simulink subsystem "InjectorPablo"  (R2020b)
settings: Solver=VariableStepAuto  StartTime=0.0  StopTime=10.0  RelTol=1e-3
model mask{centerHolesDiam=0.89e-3, edgeHolesDiam=0.63e-3}
  mask prompts: centerHolesDiam "Center holes diameter (m)"; edgeHolesDiam "Edge holes diameter (m)"
libraries: fl_lib x8, nesl_utility x2
settings Model: Creator=Edward  LastModifiedBy=Edward

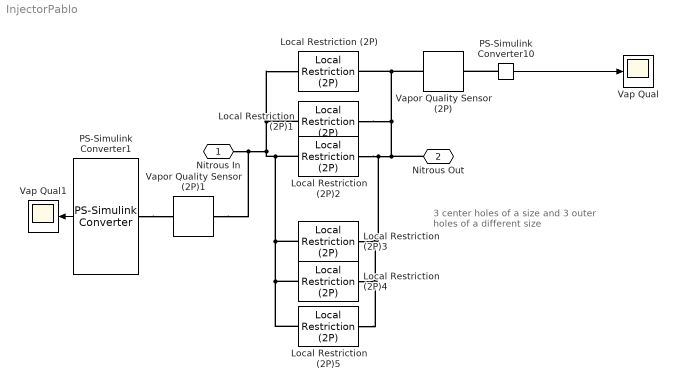
== system InjectorPablo ==
  note: 3 center holes of a size
      | and 3 outer holes of a different size
  Local Restriction (2P) : fl_lib/Two-Phase Fluid/Elements/Local Restriction (2P)  restriction_area=0.25.*pi.*centerHolesDiam.^2 m^2  area=Sim.preInjectorPipe.crossSection m^2  Cd=0.64  B_lam=0.999
      settings: SourceProductBaseCode=SS  InternalSimscapePortConfiguration="{\"Bottom\":[],\"Left\":[{\"id\":\"A\",\"label\":\"A\",\"type\":\"foundation.two_phase_fluid.two_phase_fluid\"}],\"Right\":[{\"id\":\"B\",\"label\":\"B\",\"type\":\"foundation.two_phase_fluid.two_phase_fluid\"}],\"Top\":[]}"
  Local Restriction (2P)1 : fl_lib/Two-Phase Fluid/Elements/Local Restriction (2P)  restriction_area=0.25.*pi.*centerHolesDiam.^2 m^2  area=Sim.preInjectorPipe.crossSection m^2  Cd=0.64  B_lam=0.999
      settings: SourceProductBaseCode=SS  InternalSimscapePortConfiguration="{\"Bottom\":[],\"Left\":[{\"id\":\"A\",\"label\":\"A\",\"type\":\"foundation.two_phase_fluid.two_phase_fluid\"}],\"Right\":[{\"id\":\"B\",\"label\":\"B\",\"type\":\"foundation.two_phase_fluid.two_phase_fluid\"}],\"Top\":[]}"
  Local Restriction (2P)2 : fl_lib/Two-Phase Fluid/Elements/Local Restriction (2P)  restriction_area=0.25.*pi.*centerHolesDiam.^2 m^2  area=Sim.preInjectorPipe.crossSection m^2  Cd=0.64  B_lam=0.999
      settings: SourceProductBaseCode=SS  InternalSimscapePortConfiguration="{\"Bottom\":[],\"Left\":[{\"id\":\"A\",\"label\":\"A\",\"type\":\"foundation.two_phase_fluid.two_phase_fluid\"}],\"Right\":[{\"id\":\"B\",\"label\":\"B\",\"type\":\"foundation.two_phase_fluid.two_phase_fluid\"}],\"Top\":[]}"
  Local Restriction (2P)3 : fl_lib/Two-Phase Fluid/Elements/Local Restriction (2P)  restriction_area=0.25.*pi.*edgeHolesDiam.^2 m^2  area=Sim.preInjectorPipe.crossSection m^2  Cd=0.64  B_lam=0.999
      settings: SourceProductBaseCode=SS  InternalSimscapePortConfiguration="{\"Bottom\":[],\"Left\":[{\"id\":\"A\",\"label\":\"A\",\"type\":\"foundation.two_phase_fluid.two_phase_fluid\"}],\"Right\":[{\"id\":\"B\",\"label\":\"B\",\"type\":\"foundation.two_phase_fluid.two_phase_fluid\"}],\"Top\":[]}"
  Local Restriction (2P)4 : fl_lib/Two-Phase Fluid/Elements/Local Restriction (2P)  restriction_area=0.25.*pi.*edgeHolesDiam.^2 m^2  area=Sim.preInjectorPipe.crossSection m^2  Cd=0.64  B_lam=0.999
      settings: SourceProductBaseCode=SS  InternalSimscapePortConfiguration="{\"Bottom\":[],\"Left\":[{\"id\":\"A\",\"label\":\"A\",\"type\":\"foundation.two_phase_fluid.two_phase_fluid\"}],\"Right\":[{\"id\":\"B\",\"label\":\"B\",\"type\":\"foundation.two_phase_fluid.two_phase_fluid\"}],\"Top\":[]}"
  Local Restriction (2P)5 : fl_lib/Two-Phase Fluid/Elements/Local Restriction (2P)  restriction_area=0.25.*pi.*edgeHolesDiam.^2 m^2  area=Sim.preInjectorPipe.crossSection m^2  Cd=0.64  B_lam=0.999
      settings: SourceProductBaseCode=SS  InternalSimscapePortConfiguration="{\"Bottom\":[],\"Left\":[{\"id\":\"A\",\"label\":\"A\",\"type\":\"foundation.two_phase_fluid.two_phase_fluid\"}],\"Right\":[{\"id\":\"B\",\"label\":\"B\",\"type\":\"foundation.two_phase_fluid.two_phase_fluid\"}],\"Top\":[]}"
  PS-Simulink Converter1 : nesl_utility/PS-Simulink Converter  PhysicalDomain=network_engine_domain  SubClassName=ps_output  LeftPortType=input  RightPortType=output  PseudoPeriodic=off  Frequencies=[]  Unit=inherit  AffineConversion=off
  PS-Simulink Converter10 : nesl_utility/PS-Simulink Converter  PhysicalDomain=network_engine_domain  SubClassName=ps_output  LeftPortType=input  RightPortType=output  PseudoPeriodic=off  Frequencies=[]  Unit=inherit  AffineConversion=off
  Vap Qual : Scope
  Vap Qual1 : Scope
  Vapor Quality Sensor (2P) : fl_lib/Two-Phase Fluid/Sensors/Vapor Quality Sensor (2P)  vapor_fraction_spec=foundation.enum.vapor_fraction_spec.quality
      settings: SourceProductBaseCode=SS  InternalSimscapePortConfiguration="{\"Bottom\":[],\"Left\":[{\"id\":\"A\",\"label\":\"A\",\"type\":\"foundation.two_phase_fluid.two_phase_fluid\"}],\"Right\":[{\"id\":\"X\",\"label\":\"X\",\"type\":\"output\"}],\"Top\":[]}"
  Vapor Quality Sensor (2P)1 : fl_lib/Two-Phase Fluid/Sensors/Vapor Quality Sensor (2P)  vapor_fraction_spec=foundation.enum.vapor_fraction_spec.quality
      settings: SourceProductBaseCode=SS  InternalSimscapePortConfiguration="{\"Bottom\":[],\"Left\":[{\"id\":\"A\",\"label\":\"A\",\"type\":\"foundation.two_phase_fluid.two_phase_fluid\"}],\"Right\":[{\"id\":\"X\",\"label\":\"X\",\"type\":\"output\"}],\"Top\":[]}"
  Nitrous In : PMIOPort  Side=Left
  Nitrous Out : PMIOPort  Port=2  Side=Right
  wires:
  PS-Simulink Converter10/1 -> Vap Qual/1
  PS-Simulink Converter1/1 -> Vap Qual1/1
  connections:
  Local Restriction (2P)4/RConn1 -- Local Restriction (2P)/RConn1 -- Vapor Quality Sensor (2P)/LConn1 -- Local Restriction (2P)1/RConn1 -- Nitrous Out/RConn1 -- Local Restriction (2P)2/RConn1 -- Local Restriction (2P)3/RConn1 -- Local Restriction (2P)5/RConn1
  Local Restriction (2P)4/LConn1 -- Vapor Quality Sensor (2P)1/LConn1 -- Nitrous In/RConn1 -- Local Restriction (2P)/LConn1 -- Local Restriction (2P)1/LConn1 -- Local Restriction (2P)2/LConn1 -- Local Restriction (2P)3/LConn1 -- Local Restriction (2P)5/LConn1
  PS-Simulink Converter10/LConn1 -- Vapor Quality Sensor (2P)/RConn1
  PS-Simulink Converter1/LConn1 -- Vapor Quality Sensor (2P)1/RConn1
